simulink model "Nivel_R1_R2_2018"  (R2018a)
settings: Solver=VariableStepAuto  StartTime=0.0  StopTime=700  RelTol=1e-3
values from neighbouring files (symbols this model uses):
  a1 = q*(100/6)./(sqrt(2*981*h10))    [init.m]    (also in init_quarta.m)
  a2 = q*(100/6)./(sqrt(2*981*h20))    [init.m]    (also in init_quarta.m)
  h10 = Z(2,ii)    [init.m]    (also in init_quarta.m)
  h20 = Z(3,ii)    [init.m]    (also in init_quarta.m)
undefined symbols (not defined in the file or in its folder): Ar, qs
settings Model: Creator=celsojosemunaro  LastModifiedBy=celsojosemunaro
settings DataIOCC: ReturnWorkspaceOutputs=on
settings SFSimCC: SimUseLocalCustomCode=on
settings RTWCC: RTWUseLocalCustomCode=on

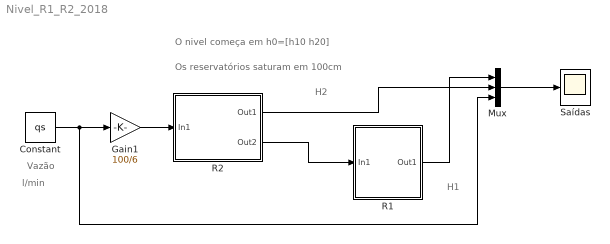
== system Nivel_R1_R2_2018 ==
  note: Vazão
  note: Os reservatórios saturam em 100cm
  note: H1
  note: H2
  note: O nivel começa em h0=[h10 h20]
  note: l/min
  Constant : Constant  Value=qs
  Gain1 : Gain  Gain=100/6
  Mux : Mux  Inputs=3
  R1 : Subsystem
  R2 : Subsystem
  Saídas : Scope
  wires:
  Mux/1 -> Saídas/1
  Gain1/1 -> R2/1(In1)
  R2/1(Out1) -> Mux/2
  R2/2(Out2) -> R1/1(In1)
  R1/1(Out1) -> Mux/1
  Constant/1 -> Mux/3, Gain1/1

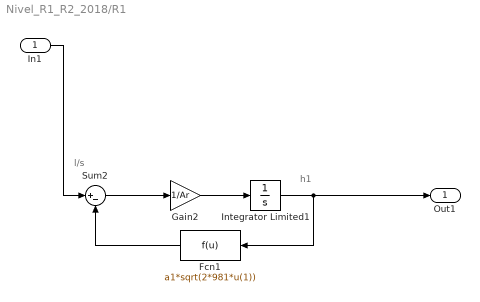
== system Nivel_R1_R2_2018/R1 ==
  note: l/s
  note: h1
  In1 : Inport
  Fcn1 : Fcn  Expr=a1*sqrt(2*981*u(1))
  Gain2 : Gain  Gain=1/Ar
  Integrator Limited1 : Integrator  InitialCondition=h10  LimitOutput=on  UpperSaturationLimit=100  LowerSaturationLimit=0
  Sum2 : Sum  Inputs=|+-
  Out1 : Outport
  wires:
  In1/1 -> Sum2/1
  Gain2/1 -> Integrator Limited1/1
  Integrator Limited1/1 -> Out1/1, Fcn1/1
  Sum2/1 -> Gain2/1
  Fcn1/1 -> Sum2/2

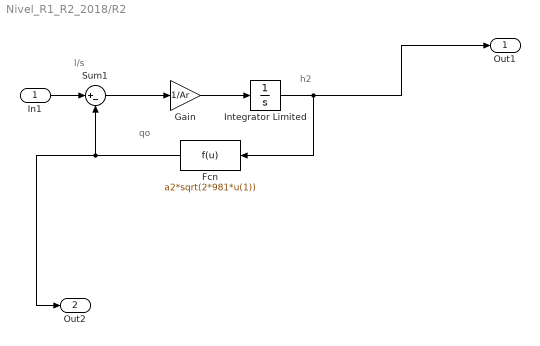
== system Nivel_R1_R2_2018/R2 ==
  note: l/s
  note: h2
  note: qo
  In1 : Inport
  Fcn : Fcn  Expr=a2*sqrt(2*981*u(1))
  Gain : Gain  Gain=1/Ar
  Integrator Limited : Integrator  InitialCondition=h20  LimitOutput=on  UpperSaturationLimit=100  LowerSaturationLimit=0
  Sum1 : Sum  Inputs=|+-
  Out1 : Outport
  Out2 : Outport  Port=2
  wires:
  Gain/1 -> Integrator Limited/1
  Sum1/1 -> Gain/1
  Fcn/1 -> Out2/1, Sum1/2
  In1/1 -> Sum1/1
  Integrator Limited/1 -> Out1/1, Fcn/1
